simulink model "control_design"  (R2018b)
settings: Solver=FixedStepAuto  StartTime=0.0  StopTime=20  FixedStep=.02  RelTol=1e-3
libraries: simulink x8
settings Model: Creator=Tyler  LastModifiedBy=Tyler

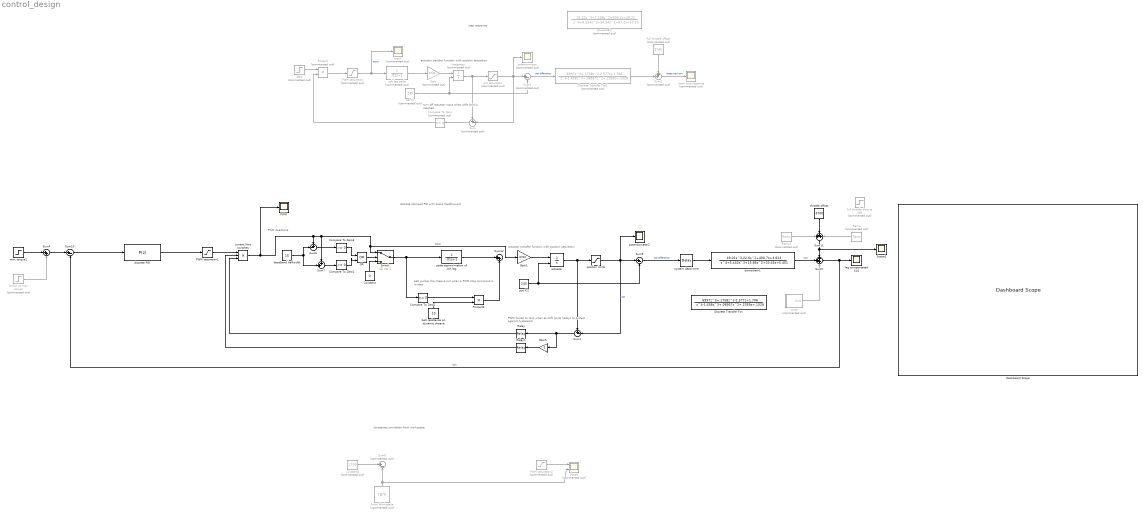
== system control_design ==
  note: PWM deadzone
  note: turn off actuator input
      | when shift limit is reached
  note: actuator transfer function with position saturation
  note: PWM forced to zero when at shift limits
      |  (relays to protect against hysteresis)
  note: actuator transfer function with position saturation
  note: belt pushes the sheave out when a PWM
      | stop command is written
  note: step response
  note: discrete clamped PID with brake feedforward
  note: timeseries simulation from workspace
  Compare To Zero : simulink/Logic and Bit Operations/Compare To Zero  Commented=on  relop===  OutDataTypeStr=boolean
  Compare To Zero1 : simulink/Logic and Bit Operations/Compare To Zero  relop=<=  OutDataTypeStr=boolean
  Compare To Zero2 : simulink/Logic and Bit Operations/Compare To Zero  relop===  OutDataTypeStr=boolean
  Compare To Zero3 : simulink/Logic and Bit Operations/Compare To Zero  relop=>=  OutDataTypeStr=boolean
  Constant : Constant  Value=0
  Constant1 : Constant  Commented=on  Value=2700
  Dashboard Scope : DashboardScope  WebBlockId=384
  Discrete Transfer Fcn : DiscreteTransferFcn  Numerator=[.6997 .1758 -2.577 1.706]  Denominator=[1 -1.458 .08957 .2359 .1328]  SampleTime=.02
  Discrete Transfer Fcn1 : DiscreteTransferFcn  Commented=on  Numerator=[.6997 .1758 -2.577 1.706]  Denominator=[1 -1.458 .08957 .2359 .1328]  SampleTime=.02
  From Workspace : FromWorkspace  Commented=on  VariableName=rpm  SampleTime=.02  Interpolate=off  OutputAfterFinalValue=Holding final value
  Gain : Gain  Commented=on  Gain=.0743
  Gain1 : Gain  Gain=.0742
  Gain5 : Gain  Gain=-1
  Integrator : Integrator  Commented=on  InitialConditionSource=external  InitialCondition=762
  OR : Logic  Operator=OR  IconShape=distinctive  AllPortsSameDT=off  OutDataTypeStr=boolean
  PWM : Scope
  PWM saturation : Saturate  Commented=on  UpperLimit=500  LowerLimit=-500
  PWM saturation1 : Saturate  UpperLimit=500  LowerLimit=-500
  PWM saturation2 : Saturate  Commented=on  UpperLimit=500  LowerLimit=-500
  Product : Product  Commented=on
  Product3 : Product
  Ramp : simulink/Sources/Ramp  Commented=on  slope=3700  start=0  InitialOutput=0
  Ramp1 : simulink/Sources/Ramp  Commented=on  slope=-3700  start=1  InitialOutput=0
  Relay : Relay  OnSwitchValue=1  OffSwitchValue=0  OnOutputValue=0  OffOutputValue=1
  Relay1 : Relay  OnSwitchValue=1  OffSwitchValue=0  OnOutputValue=0  OffOutputValue=1
  Scope : Scope  Commented=on  NumInputPorts=2
  Scope1 : Scope
  Step : Step  Commented=on  Time=0  After=-500  SampleTime=0
  Sum : Sum  Commented=on  Inputs=+-|
  Sum1 : Sum  Inputs=+-|
  Sum10 : Sum  Inputs=|+-
  Sum11 : Sum  Inputs=+++
  Sum12 : Sum  Inputs=|++
  Sum2 : Sum  Commented=on  Inputs=++|
  Sum3 : Sum  Commented=on  Inputs=|+-
  Sum4 : Sum  Inputs=|++
  Sum5 : Sum  Inputs=+++
  Sum6 : Sum  Inputs=+-|
  Sum7 : Sum  Inputs=++|
  Sum8 : Sum  Commented=on  Inputs=|+-
  Sum9 : Sum  Inputs=|+-
  Switch : Switch  Threshold=1
  actuator : Integrator  InitialConditionSource=external  InitialCondition=762  UpperSaturationLimit=460  LowerSaturationLimit=146
  belt resistance on dynamic sheave : Constant  Value=10
  current limit switches : Product  Inputs=3
  deadband halfwidth : Constant  Value=15
  discrete PID : simulink/Continuous/PID Controller  Controller=P  Form=Parallel  TimeDomain=Discrete-time  SampleTime=.02  IntegratorMethod=Trapezoidal  FilterMethod=Forward Euler  ControllerParametersSource=internal  P=100  I=2.744  D=.626  UseFilter=on  N=100  TunerSelectOption=Transfer Function Based (PID Tuner App)  InitialConditionSource=internal  InitialConditionForIntegrator=0  InitialConditionForFilter=0  DifferentiatorICPrevScaledInput=0  ExternalReset=none  TrackingMode=off  Kt=1  LimitOutput=on  UpperSaturationLimit=500  LowerSaturationLimit=-500  LinearizeAsGain=on  AntiWindupMode=clamping  Kb=1  POutMin=[]  POutMax=[]  IOutMin=[]  IOutMax=[]  DOutMin=[]  DOutMax=[]  NOutMin=[]  NOutMax=[]  SumOutMin=[]  SumOutMax=[]  SaturationOutMin=[]  SaturationOutMax=[]  PParamMin=[]  PParamMax=[]  IParamMin=[]  IParamMax=[]  DParamMin=[]  DParamMax=[]  NParamMin=[]  NParamMax=[]  KbParamMin=[]  KbParamMax=[]  KtParamMin=[]  KtParamMax=[]  KbOutMin=[]  KbOutMax=[]  KtOutMin=[]  KtOutMax=[]  IntegratorOutMin=[]  IntegratorOutMax=[]  FilterOutMin=[]  FilterOutMax=[]  SumI1OutMin=[]  SumI1OutMax=[]  SumI2OutMin=[]  SumI2OutMax=[]  SumI3OutMin=[]  SumI3OutMax=[]  SumI4OutMin=[]  SumI4OutMax=[]  SumDOutMin=[]  SumDOutMax=[]  DifferentiatorOutMin=[]  DifferentiatorOutMax=[]  FilterDiffOutCoefMin=[]  FilterDiffOutCoefMax=[]  ReciprocalOutMin=[]  ReciprocalOutMax=[]  SumDenOutMin=[]  SumDenOutMax=[]  SumNumOutMin=[]  SumNumOutMax=[]  DivideOutMin=[]  DivideOutMax=[]  IntegratorContinuousStateAttributes=''  IntegratorStateMustResolveToSignalObject=off  IntegratorRTWStateStorageClass=Auto  FilterContinuousStateAttributes=''  FilterStateMustResolveToSignalObject=off  FilterRTWStateStorageClass=Auto  ParallelPVariant=InternalParameters  IdealPVariant=Disabled  IVariant=Disabled  DVariant=Disabled  IntegratorVariant=Disabled  SatVariant=Enabled  AWVariant=Disabled  PCopyVariant=Disabled  TRVariant=Disabled  FdbkBlocksVariant=Forward  IdealPFdbkVariant=Disabled  SatFdbkVariant=Disabled  DerivativeFilterVariant=Disabled  NVariant=Disabled  NCopyVariant=Disabled_SignalSpec  FilterICVariant=Disabled  IntegratorICVariant=Disabled  ExternalResetVariant=Disabled  TRSumVariant=Passthrough  SumFdbkVariant=Disabled  SumVariant=Passthrough_P
  full throttle drop to idle : Step  Commented=on  Time=5  After=-2200.  SampleTime=0
  full throttle offset : Constant  Commented=on  Value=3700
  input : Scope  Commented=on
  lag compensated CLS : Scope
  max torque1 : Step  Time=0  After=2700  SampleTime=0
  noise : Subsystem  Commented=on
  open loop response : Scope  Commented=on
  pade approximation of zoh lag : TransferFcn  Denominator=[.01 1]
  position limits : Saturate  UpperLimit=245  LowerLimit=165
  pot IC : Constant  Commented=on  Value=245
  pot IC2 : Constant  Value=245
  pot saturation : Saturate  Commented=on  UpperLimit=460  LowerLimit=146
  potentiometer : Scope  Commented=on
  potentiometer2 : Scope
  powertrain : TransferFcn  Commented=on  Numerator=[35.02 7.238 509.2 49.21]  Denominator=[1 6.234 54.54 87.2 53.23]
  powertrain1 : TransferFcn  Numerator=[49.01 -22.6 400.7 3.623]  Denominator=[1 5.432 15.86 33.45 5.401]
  switch to max power : Step  Commented=on  Time=4  After=700  SampleTime=0
  system dead time : TransportDelay  DelayTime=9*.02
  throttle offset : Constant  Value=3700
  zoh lag pade : TransferFcn  Commented=on  Denominator=[.01 1]
  wires:
  Sum2/1 -> open loop response/1  "measured rpm"
  full throttle offset/1 -> Sum2/1
  Step/1 -> Product/1
  PWM saturation/1 -> input/1, zoh lag pade/1  "PWM"
  Sum5/1 -> Sum10/2, lag compensated CLS/1  "rpm"
  Sum9/1 -> system dead time/1  "pot difference"
  Sum11/1 -> Scope1/1, Sum5/1
  Product3/1 -> Sum12/2
  belt resistance on dynamic sheave/1 -> Product3/2
  Compare To Zero2/1 -> Product3/1
  Relay1/1 -> current limit switches/2
  Relay/1 -> current limit switches/3
  position limits/1 -> potentiometer2/1, Sum1/2, Sum9/1  "pot"
  Gain5/1 -> Relay1/1
  Sum1/1 -> Gain5/1, Relay/1
  pot IC/1 -> Sum3/2, Integrator/2
  zoh lag pade/1 -> Gain/1
  Gain/1 -> Integrator/1
  Compare To Zero/1 -> Product/2
  pot saturation/1 -> Sum3/1, Sum/2, potentiometer/1
  Integrator/1 -> pot saturation/1, Sum/1
  Sum/1 -> Compare To Zero/1
  Sum4/1 -> Sum10/1
  switch to max power/1 -> Sum4/2
  max torque1/1 -> Sum4/1
  noise/1(Out1) -> Sum5/3
  Gain1/1 -> actuator/1
  pot IC2/1 -> Sum9/2, actuator/2
  pade approximation of zoh lag/1 -> Sum12/1
  Product/1 -> PWM saturation/1
  Sum6/1 -> Compare To Zero3/1
  Compare To Zero1/1 -> OR/2
  OR/1 -> Switch/2
  Constant/1 -> Switch/3
  Sum7/1 -> Compare To Zero1/1
  deadband halfwidth/1 -> Sum7/2, Sum6/2
  Compare To Zero3/1 -> OR/1
  Switch/1 -> Compare To Zero2/1, pade approximation of zoh lag/1
  current limit switches/1 -> PWM/1, Sum6/1, Sum7/1, Gain1/1, Switch/1  "PWM"
  actuator/1 -> position limits/1, Sum1/1
  PWM saturation2/1 -> Scope/1
  From Workspace/1 -> Sum8/2, Scope/2
  Constant1/1 -> Sum8/1
  Ramp1/1 -> Sum11/1
  throttle offset/1 -> Sum11/2
  Ramp/1 -> Sum11/3
  PWM saturation1/1 -> current limit switches/1
  Discrete Transfer Fcn1/1 -> Sum2/2
  Sum3/1 -> Discrete Transfer Fcn1/1  "pot difference"
  system dead time/1 -> powertrain1/1
  powertrain1/1 -> Sum5/2  "rpm"
  Sum10/1 -> discrete PID/1
  discrete PID/1 -> PWM saturation1/1

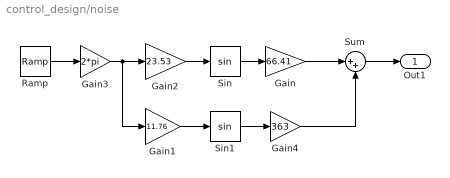
== system control_design/noise ==
  Gain : Gain  Gain=66.41
  Gain1 : Gain  Gain=11.76
  Gain2 : Gain  Gain=23.53
  Gain3 : Gain  Gain=2*pi
  Gain4 : Gain  Gain=363
  Ramp : simulink/Sources/Ramp  slope=1  start=0  InitialOutput=0
  Sin : Trigonometry
  Sin1 : Trigonometry
  Sum : Sum  Inputs=|++
  Out1 : Outport
  wires:
  Ramp/1 -> Gain3/1
  Gain3/1 -> Gain1/1, Gain2/1
  Gain1/1 -> Sin1/1
  Gain2/1 -> Sin/1
  Sin/1 -> Gain/1
  Sin1/1 -> Gain4/1
  Sum/1 -> Out1/1
  Gain/1 -> Sum/1
  Gain4/1 -> Sum/2
